simulink model "Induction_Motor"  (R2015a)
settings: Solver=FixedStepDiscrete  StartTime=0.0  StopTime=3  FixedStep=Ts  RelTol=1e-3
InitFcn:
  | Ts=1e-5;
values from neighbouring files (symbols this model uses):
  Mech_Load = 0.0    (= 0)    [runDistSim.m]    (also in run_all_dist_induction.m = [0.20, 0.80]*NominalTorque)
  Speed_Target = 1200    [runDistSim.m]    (also in run_all_dist_induction.m = 2240)
undefined symbols (not defined in the file or in its folder): ctrl_sat
libraries: powerlib x17, powerlib_extras x3, simulink x1, AC6DriveInternalModels x1
settings Model: Creator=Mademlis  LastModifiedBy=Savvas
settings DataIOCC: SignalLoggingSaveFormat=ModelDataLogs
settings OptimizationCC: ExpressionDepthLimit=2147483647
settings DebuggingCC: UnderspecifiedInitializationDetection=Classic  MergeDetectMultiDrivingBlocksExec=none  SolverPrmCheckMsg=warning  FcnCallInpInsideContextMsg=EnableAllAsWarning  StateNameClashWarn=warning

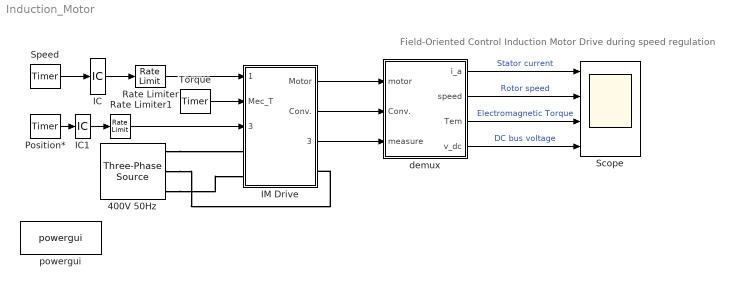
== system Induction_Motor ==
  note: Field-Oriented Control Induction Motor Drive during speed regulation
  400V 50Hz : powerlib/Electrical Sources/Three-Phase Source  Voltage=400  PhaseAngle=0  Frequency=50  InternalConnection=Yg  SpecifyImpedance=off  Resistance=0.02  Inductance=0.05e-3  ShortCircuitLevel=100e6  BaseVoltage=25e3  XRratio=7  BusType=swing  Pref=0  Qref=0  Qmin=-inf  Qmax=inf
  IC : InitialCondition  Value=0
  IC1 : InitialCondition  Value=0
  IM Drive : Subsystem
  Position* : powerlib_extras/Control  Blocks/Timer  t=[0 0.9]  e=[400 400]
  Rate Limiter : RateLimiter  RisingSlewLimit=600000  FallingSlewLimit=-600000  LinearizeAsGain=off
  Rate Limiter1 : RateLimiter  RisingSlewLimit=5000  FallingSlewLimit=-5000  LinearizeAsGain=off
  Scope : Scope  NumInputPorts=4
      settings: TimeRange=1.5  YMin=-28.89936~-296.83949~-32.87981~-120.93965  YMax=31.56272~1411.46172~57.70988~1089.39505  SaveName=simout  Decimation=25
  Speed : powerlib_extras/Control  Blocks/Timer  t=[0 0.1]  e=[0 Speed_Target]
  Torque : powerlib_extras/Control  Blocks/Timer  t=[0 0.6]  e=[0 Mech_Load]*10
  demux : Subsystem
  powergui : powerlib/powergui  Priority=2  SimulationMode=Discrete  SolverType=Tustin  SampleTime=Ts  frequency=60  SPID=off  DisableSnubberDevices=off  DisableRonSwitches=off  DisableVfSwitches=off  SwTol=0  DisplayEquations=off  Interpol=off  methode=off  Ts=0  FunctionMessages=off  echomessages=off  HookPort=off  EnableUseOfTLC=off  x0status=blocks  frequencyindice=50  Pbase=100e6  ErrMax=1e-4  Iterations=50  UnitsV=kV  UnitsW=MW  buscounter=0  RestoreLinks=warning  ResistiveCurrentMeasurement=off  Frange=[0:2:500]  Ylog=off  Xlog=on  ShowGrid=off  save=off  variable=ZData  structure=simout  ZoomFFT=on  StartTime=0.05  cycles=7  DisplayStyle=1  fundamental=60  FreqAxis=off  MaxFrequency=20000  frequencyindicesteady=1  RmsSteady=1  display=off
  wires:
  demux/1(i_a) -> Scope/1  "Stator current"
  demux/3(Tem) -> Scope/3  "Electromagnetic Torque"
  demux/4(v_dc) -> Scope/4  "DC bus voltage"
  demux/2(speed) -> Scope/2  "Rotor speed"
  Torque/1 -> IM Drive/2(Mec_T)
  Position*/1 -> IC1/1
  Rate Limiter/1 -> IM Drive/1(Speed*)
  Rate Limiter1/1 -> IM Drive/3(Position*)
  IC1/1 -> Rate Limiter1/1
  IM Drive/1(Motor) -> demux/1(motor)
  IM Drive/2(Conv.) -> demux/2(Conv.)
  IM Drive/3(measure) -> demux/3(measure)
  Speed/1 -> IC/1
  IC/1 -> Rate Limiter/1
  connections:
  400V 50Hz/RConn3 -- IM Drive/LConn2
  400V 50Hz/RConn1 -- IM Drive/LConn1
  400V 50Hz/RConn2 -- IM Drive/RConn1

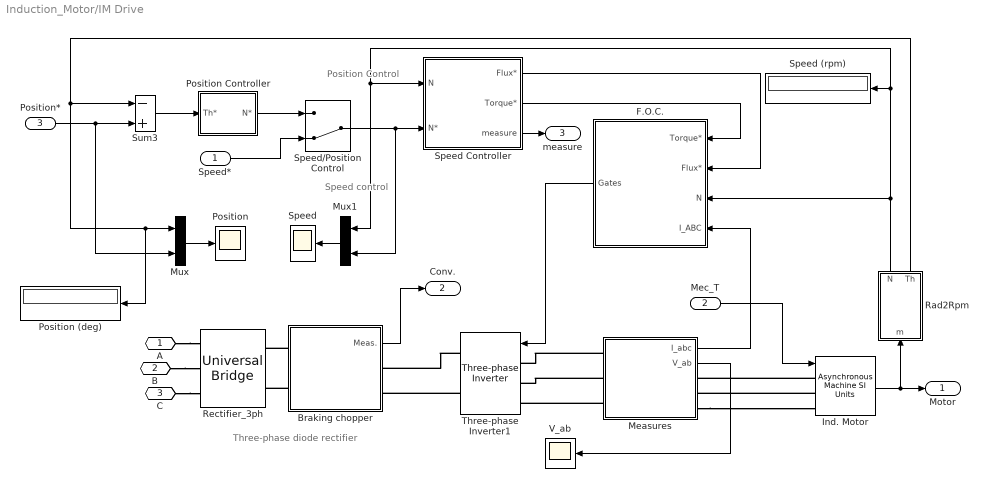
== system Induction_Motor/IM Drive ==
  note: Speed
      | control
  note: Position
      |  Control
  note: Three-phase
      | diode rectifier
  Speed* : Inport
  Mec_T : Inport  Port=2
  Position* : Inport  Port=3
  Braking chopper : Subsystem  mask(Braking chopper){chopa=650, chopd=530, freq_chop=1000, cap_bus=1500e-6, br=30}
      mask prompts: chopa "Chopper activation voltage (V)"; chopd "Chopper shutdown voltage (V)"; freq_chop "Braking chopper frequency (Hz)"; cap_bus "DC bus capacitance (F)"; br "Braking resistance (ohms)"
      mask help: This block implements a DC link between the rectifier and the inverter. It also contains a DC bus integrated braking chopper. The braking resistor must be set properly to avoid oscillation.
      mask init:
      | [X1,X1m,X2,X2m,X3,X4,Y1,Y1m,Y2,Y2m,Y3,Y4,color1,color2]=spsdrivelogo;
      mask Display:
      | patch([X1 X1m],[Y1 Y1m],color1);
      | patch(X3,Y3,color2);
      | plot([X1 X1m X2 X2m X3 X4],[Y1 Y1m Y2 Y2m Y3 Y4]);
  F.O.C. : Subsystem  mask(FOC){in_flux=0.85, Lm=0.50, Lls=0.027, Rr=3.2, Llr=0.027, p=2, Tvect=50e-6}
      mask prompts: in_flux "Initial machine flux (Wb)"; Lm "Motor mutual inductance (H)"; Lls "Motor stator Leakage inductance (H)"; Rr "Motor rotor resistance (ohms)"; Llr "Motor rotor leakage inductance (H)"; p "Motor pairs of poles"; Tvect "Vector control sampling time (s)"
      mask help: This block implements a field oriented controller.
      mask init:
      | Lr=Lm+Llr;
      | Ls=Lm+Lls;
      | [X1,X1m,X2,X2m,X3,X4,Y1,Y1m,Y2,Y2m,Y3,Y4,color1,color2]=spsdrivelogo;
      mask Display:
      | patch([X1 X1m],[Y1 Y1m],color1);
      | patch(X3,Y3,color2);
      | plot([X1 X1m X2 X2m X3 X4],[Y1 Y1m Y2 Y2m Y3 Y4]);
  Ind. Motor : powerlib/Machines/Asynchronous Machine SI Units  RotorType=Squirrel-cage  PresetModel=No  MechanicalLoad=Torque Tm  ShowDetailedParameters=on  ReferenceFrame=Rotor  Units=SI  MeasurementBus=off  NominalParameters=[2040 380 50]  Stator=[5.8 0.027]  Rotor=[3.2 0.027]  Cage1=[ 0.022 0.226/377]  Cage2=[ 0.022 0.226/377]  Lm=0.5  Mechanical=[0.047 0 2]  PolePairs=2  InitialConditions=[1 0 0 0 0 0 0 0]  SimulateSaturation=off  Saturation=[14.03593122, 27.81365428, 53.79336849, 72.68890987, 97.98006896, 148.6815601, 215.7428561, 302.9841135, 428.7778367 ; 230, 322, 414, 460, 506, 552, 598, 644, 690]  LoadFlowParameters=1492000  TsPowergui=0  TsBlock=-1  IterativeModel=Forward Euler  Pmec=1500
  Measures : Subsystem
  Mux : Mux  Inputs=2
  Mux1 : Mux  Inputs=2
  Position : Scope
      settings: YMin=-333.29346  YMax=2985.49263  SaveName=Angle
  Position (deg) : Display
  Position Controller : Subsystem  mask{Kp_th=2, T_position=5e-3}
      mask prompts: Kp_th "Proportional gain"; T_position "Controllersampling time (s)"
  Rad2Rpm : Subsystem
  Rectifier_3ph : powerlib/Power Electronics/Universal Bridge  Arms=3  SnubberResistance=10e3  SnubberCapacitance=20e-9  Device=Diodes  Ron=1e-3  Lon=0  ForwardVoltages="[  0,  0  ]"  ForwardVoltage=1.3  GTOparameters=[ 10e-6, 20e-6 ]  IGBTparameters=[ 1e-6 , 2e-6 ]  Measurements=All voltages and currents  Measurements_2=None  converterType=Rectifier
  Speed : Scope
      settings: TimeRange=1  YMin=-400  YMax=1400  SaveName=Speed_ref
  Speed (rpm) : Display
  Speed Controller : Subsystem  mask(Speed controller){kp=0.15, ki=0.0455, fc=50, ctrl_sat=[-30, 30], p=2, nf=0.85, Tsc=5e-3}
      mask prompts: kp "Proportional gain"; ki "Integral gain"; fc "Speed measurement - low-pass filter cutoff frequency (Hz)"; ctrl_sat "Controller output torque saturation (N.m) [negative,positive]"; p "Motor pairs of poles"; nf "Machine nominal flux (Wb)"; Tsc "Controller sampling time (s)"
      mask help: This block implements a PI speed regulator.
      mask init:
      | [X1,X1m,X2,X2m,X3,X4,Y1,Y1m,Y2,Y2m,Y3,Y4,color1,color2]=spsdrivelogo;
      mask Display:
      | patch([X1 X1m],[Y1 Y1m],color1);
      | patch(X3,Y3,color2);
      | plot([X1 X1m X2 X2m X3 X4],[Y1 Y1m Y2 Y2m Y3 Y4]);
  Speed/Position Control : ManualSwitch  CurrentSetting=0
  Sum3 : Sum  Inputs=-+  SaturateOnIntegerOverflow=on  InputSameDT=on  OutDataTypeStr=Inherit: Same as first input
  Three-phase Inverter1 : AC6DriveInternalModels/Three-phase Inverter  Arms=3  SnubberResistance=5000  SnubberCapacitance=inf  Device=IGBT / Diodes  Ron=1e-3  Lon=0  ForwardVoltages=[0.8,0.8]  ForwardVoltage=0  GTOparameters=[0,0]  IGBTParameters=[1e-6,2e-6]  Measurements=All voltages and currents  converterType=Inverter  SourceFrequency=60  dqInductances=[8.5e-3,8.5e-3]  Flux=0.175  Resistance=0.2  p=4
  V_ab : Scope
      settings: YMin=-50  YMax=50  SaveName=simout1
  A : PMIOPort  Port=1  Side=Left
  B : PMIOPort  Port=2  Side=Right
  C : PMIOPort  Port=3  Side=Left
  Motor : Outport
  Conv. : Outport  Port=2
  measure : Outport  Port=3
  wires:
  Mux1/1 -> Speed/1
  Measures/2(V_ab) -> V_ab/1
  Position*/1 -> Sum3/2, Mux/2
  Position Controller/1(N*) -> Speed/Position Control/1
  Speed/Position Control/1 -> Speed Controller/2(N*), Mux1/2
  Speed*/1 -> Speed/Position Control/2
  Sum3/1 -> Position Controller/1(Th*)
  Mux/1 -> Position/1
  Rad2Rpm/2(Th) -> Sum3/1, Mux/1, Position (deg)/1
  F.O.C./1(Gates) -> Three-phase Inverter1/1
  Braking chopper/1(Meas.) -> Conv./1
  Speed Controller/1(Flux*) -> F.O.C./2(Flux*)
  Speed Controller/3(measure) -> measure/1
  Ind. Motor/1 -> Motor/1, Rad2Rpm/1(m)
  Measures/1(I_abc) -> F.O.C./4(I_ABC)
  Speed Controller/2(Torque*) -> F.O.C./1(Torque*)
  Mec_T/1 -> Ind. Motor/1
  Rad2Rpm/1(N) -> Speed (rpm)/1, Speed Controller/1(N), Mux1/1, F.O.C./3(N)
  connections:
  C/RConn1 -- Rectifier_3ph/LConn3
  Braking chopper/LConn2 -- Rectifier_3ph/RConn2
  A/RConn1 -- Rectifier_3ph/LConn1
  Ind. Motor/LConn2 -- Measures/RConn2
  Ind. Motor/LConn1 -- Measures/RConn1
  Measures/LConn3 -- Three-phase Inverter1/LConn3
  Measures/RConn3 -- Ind. Motor/LConn3
  Three-phase Inverter1/RConn1 -- Braking chopper/RConn1
  Three-phase Inverter1/RConn2 -- Braking chopper/RConn2
  Braking chopper/LConn1 -- Rectifier_3ph/RConn1
  B/RConn1 -- Rectifier_3ph/LConn2
  Measures/LConn1 -- Three-phase Inverter1/LConn1
  Measures/LConn2 -- Three-phase Inverter1/LConn2

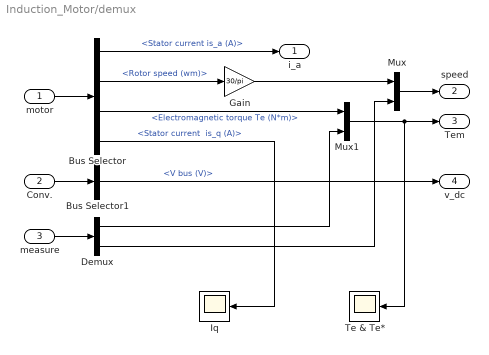
== system Induction_Motor/demux ==
  motor : Inport
  Conv. : Inport  Port=2
  measure : Inport  Port=3
  Bus Selector : BusSelector  OutputSignals="Stator measurements.Stator current is_a (A),Mechanical.Rotor speed (wm),Mechanical.Electromagnetic torque Te (N*m),Stator measurements.Stator current  is_q (A)"
  Bus Selector1 : BusSelector  OutputSignals=V bus (V)
  Demux : Demux  Outputs=2
  Gain : Gain  Gain=30/pi  SaturateOnIntegerOverflow=on  OutDataTypeStr=Inherit: Same as input  ParamDataTypeStr=Inherit: Same as input
  Iq : Scope
      settings: YMin=-50  YMax=50  SaveName=Torque1
  Mux : Mux  Inputs=2
  Mux1 : Mux  Inputs=2
  Te & Te* : Scope
      settings: YMin=-50  YMax=50  SaveName=Torque
  i_a : Outport
  speed : Outport  Port=2
  Tem : Outport  Port=3
  v_dc : Outport  Port=4
  wires:
  motor/1 -> Bus Selector/1
  Mux/1 -> speed/1
  Mux1/1 -> Tem/1, Te & Te*/1
  Bus Selector/3 -> Mux1/1  "<Electromagnetic torque Te (N*m)>"
  Bus Selector/2 -> Gain/1  "<Rotor speed (wm)>"
  Bus Selector/1 -> i_a/1  "<Stator current is_a (A)>"
  Gain/1 -> Mux/1
  Demux/2 -> Mux/2
  Demux/1 -> Mux1/2
  Conv./1 -> Bus Selector1/1
  Bus Selector1/1 -> v_dc/1  "<V bus (V)>"
  measure/1 -> Demux/1
  Bus Selector/4 -> Iq/1  "<Stator current  is_q (A)>"

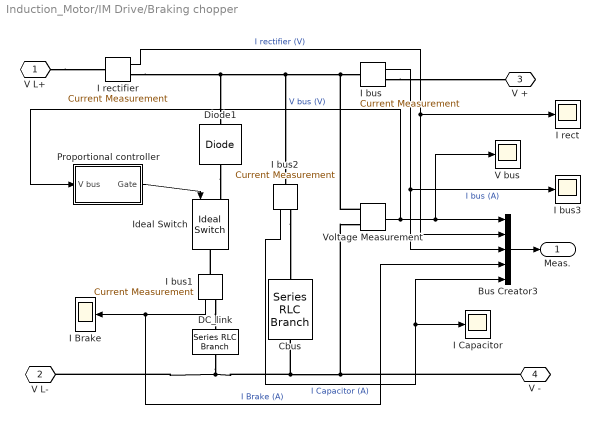
== system Induction_Motor/IM Drive/Braking chopper ==
  Bus Creator3 : BusCreator  Inputs=5
  Cbus : powerlib/Elements/Series RLC Branch  LConnTagsString=__new0  RConnTagsString=__new0  BranchType=C  Resistance=[]  Inductance=[]  SetiL0=off  InitialCurrent=0  Capacitance=cap_bus  Setx0=off  InitialVoltage=0  Measurements=None
  DC_link : powerlib/Elements/Series RLC Branch  LConnTagsString=__new0  RConnTagsString=__new0  BranchType=R  Resistance=br  Inductance=[]  SetiL0=off  InitialCurrent=0  Capacitance=[]  Setx0=off  InitialVoltage=0  Measurements=None
  Diode1 : powerlib/Power Electronics/Diode  Ron=0.01  Lon=0  Vf=0.8  IC=0  UseSnubber=off  Rs=10  Cs=10e-9  Measurements=off
  I Brake : Scope
      settings: YMin=-2.5  YMax=32.5  SaveName=I_brake
  I Capacitor : Scope
      settings: TimeRange=2  YMin=-200  YMax=200  SaveName=Ic
  I bus : powerlib/Measurements/Current Measurement  PhasorSimulation=off  OutputType=Complex  PSBequivalent=0
  I bus1 : powerlib/Measurements/Current Measurement  PhasorSimulation=off  OutputType=Complex  PSBequivalent=0
  I bus2 : powerlib/Measurements/Current Measurement  PhasorSimulation=off  OutputType=Complex  PSBequivalent=0
  I bus3 : Scope
      settings: YMin=0  YMax=950  SaveName=I_bus
  I rect : Scope
      settings: YMin=0  YMax=950  SaveName=I_rect
  I rectifier : powerlib/Measurements/Current Measurement  PhasorSimulation=off  OutputType=Complex  PSBequivalent=0
  Ideal Switch : powerlib/Power Electronics/Ideal Switch  Ron=0.01  Lon=0  IC=0  Rs=0.1  Cs=0.01e-6  Measurements=off
      settings: AttributesFormatString=\n
  Proportional controller : Subsystem
  V bus : Scope
      settings: TimeRange=2  YMin=0  YMax=950  SaveName=Vdc
  Voltage Measurement : powerlib/Measurements/Voltage Measurement  Tag=PoWeRsYsTeMmEaSuReMeNt  PhasorSimulation=off  OutputType=Complex  PSBequivalent=0
  V L+ : PMIOPort  Port=1  Side=Left
  V L- : PMIOPort  Port=2  Side=Left
  V + : PMIOPort  Port=3  Side=Right
  V - : PMIOPort  Port=4  Side=Right
  Meas. : Outport
  wires:
  Voltage Measurement/1 -> Bus Creator3/1, V bus/1, Proportional controller/1(V bus)  "V bus (V)"
  Proportional controller/1(Gate) -> Ideal Switch/1
  Bus Creator3/1 -> Meas./1
  I bus/1 -> Bus Creator3/3, I bus3/1  "I bus (A)"
  I rectifier/1 -> Bus Creator3/2, I rect/1  "I rectifier (V)"
  I bus1/1 -> I Brake/1, Bus Creator3/4  "I Brake (A)"
  I bus2/1 -> Bus Creator3/5, I Capacitor/1  "I Capacitor (A)"
  connections:
  Cbus/RConn1 -- V -/RConn1 -- Voltage Measurement/LConn2 -- V L-/RConn1 -- DC_link/RConn1
  Diode1/LConn1 -- I rectifier/RConn1 -- Voltage Measurement/LConn1 -- I bus/LConn1 -- I bus2/LConn1
  Diode1/RConn1 -- Ideal Switch/LConn1
  I bus/RConn1 -- V +/RConn1
  V L+/RConn1 -- I rectifier/LConn1
  I bus1/RConn1 -- DC_link/LConn1
  I bus1/LConn1 -- Ideal Switch/RConn1
  I bus2/RConn1 -- Cbus/LConn1

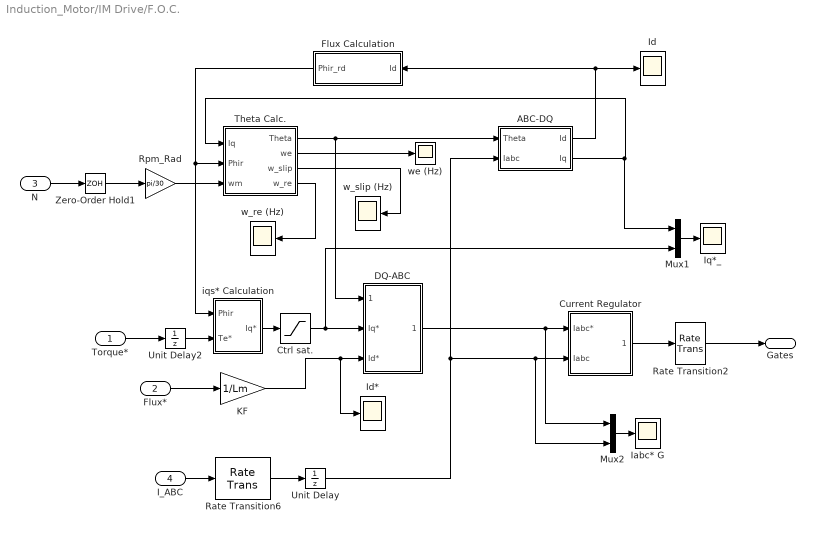
== system Induction_Motor/IM Drive/F.O.C. ==
  Torque* : Inport
  Flux* : Inport  Port=2
  N : Inport  Port=3
  I_ABC : Inport  Port=4
  ABC-DQ : Subsystem
  Ctrl sat. : Saturate  UpperLimit=26  LowerLimit=-26
  Current Regulator : Subsystem
  DQ-ABC : Subsystem
  Flux Calculation : Subsystem  mask(Flux Calcultation){}
      mask init:
      | NF=0.44572610323020e-6;
      | DF=[1 -0.99998715486734];
  Iabc* G : Scope
      settings: TimeRange=0.04  YMin=-30  YMax=30  SaveName=Iabc_G2
  Id : Scope
      settings: YMin=0  YMax=10  SaveName=Isd
  Id* : Scope
      settings: YMin=4.41347  YMax=4.87805  SaveName=Isd_ref
  Iq*_ : Scope
      settings: TimeRange=1  YMin=-20  YMax=30  SaveName=Iabc_G
  KF : Gain  Gain=1/Lm  SaturateOnIntegerOverflow=on  OutDataTypeStr=Inherit: Same as input  ParamDataTypeStr=Inherit: Same as input
  Mux1 : Mux  Inputs=2
  Mux2 : Mux  Inputs=2
  Rate Transition2 : RateTransition
  Rate Transition6 : RateTransition
  Rpm_Rad : Gain  Gain=pi/30  SaturateOnIntegerOverflow=on  OutDataTypeStr=Inherit: Same as input  ParamDataTypeStr=Inherit: Same as input
  Theta Calc. : Subsystem
  Unit Delay : UnitDelay  SampleTime=Tvect
  Unit Delay2 : UnitDelay  SampleTime=Tvect
  Zero-Order Hold1 : ZeroOrderHold  SampleTime=Tvect
  iqs* Calculation : Subsystem
  w_re (Hz) : Scope
      settings: YMin=0  YMax=100  SaveName=W_re_Hz
  w_slip (Hz) : Scope
      settings: YMin=0  YMax=100  SaveName=W_slip_Hz
  we (Hz) : Scope
      settings: YMin=-700  YMax=800  SaveName=we_Hz
  Gates : Outport
  wires:
  Mux2/1 -> Iabc* G/1
  Current Regulator/1(Pulses) -> Rate Transition2/1
  KF/1 -> DQ-ABC/3(Id*), Id*/1
  Flux*/1 -> KF/1
  iqs* Calculation/1(Iq*) -> Ctrl sat./1
  Rpm_Rad/1 -> Theta Calc./3(wm)
  ABC-DQ/1(Id) -> Id/1, Flux Calculation/1(Id)
  ABC-DQ/2(Iq) -> Mux1/1, Theta Calc./1(Iq)
  Flux Calculation/1(Phir_rd) -> iqs* Calculation/1(Phir), Theta Calc./2(Phir)
  Theta Calc./1(Theta) -> DQ-ABC/1(Theta), ABC-DQ/1(Theta)
  I_ABC/1 -> Rate Transition6/1
  Unit Delay/1 -> ABC-DQ/2(Iabc), Mux2/2, Current Regulator/2(Iabc)
  Torque*/1 -> Unit Delay2/1
  DQ-ABC/1(Iabc*) -> Mux2/1, Current Regulator/1(Iabc*)
  Rate Transition2/1 -> Gates/1
  Unit Delay2/1 -> iqs* Calculation/2(Te*)
  Rate Transition6/1 -> Unit Delay/1
  Theta Calc./2(we) -> we (Hz)/1
  Theta Calc./3(w_slip) -> w_slip (Hz)/1
  Theta Calc./4(w_re) -> w_re (Hz)/1
  Ctrl sat./1 -> Mux1/2, DQ-ABC/2(Iq*)
  Zero-Order Hold1/1 -> Rpm_Rad/1
  N/1 -> Zero-Order Hold1/1
  Mux1/1 -> Iq*_/1

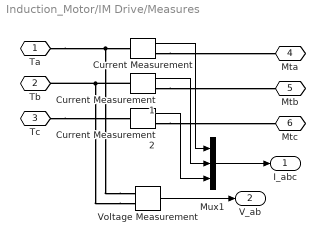
== system Induction_Motor/IM Drive/Measures ==
  Current Measurement : powerlib/Measurements/Current Measurement  Tag=PoWeRsYsTeMmEaSuReMeNt  PhasorSimulation=off  OutputType=Complex  PSBequivalent=0
  Current Measurement1 : powerlib/Measurements/Current Measurement  Tag=PoWeRsYsTeMmEaSuReMeNt  PhasorSimulation=off  OutputType=Complex  PSBequivalent=0
  Current Measurement2 : powerlib/Measurements/Current Measurement  Tag=PoWeRsYsTeMmEaSuReMeNt  PhasorSimulation=off  OutputType=Complex  PSBequivalent=0
  Mux1 : Mux  Inputs=3
  Voltage Measurement : powerlib/Measurements/Voltage Measurement  PhasorSimulation=off  OutputType=Complex  PSBequivalent=0
  Ta : PMIOPort  Port=1  Side=Left
  Tb : PMIOPort  Port=2  Side=Left
  Tc : PMIOPort  Port=3  Side=Left
  Mta : PMIOPort  Port=4  Side=Right
  Mtb : PMIOPort  Port=5  Side=Right
  Mtc : PMIOPort  Port=6  Side=Right
  I_abc : Outport
  V_ab : Outport  Port=2
  wires:
  Mux1/1 -> I_abc/1
  Current Measurement1/1 -> Mux1/2
  Current Measurement/1 -> Mux1/1
  Current Measurement2/1 -> Mux1/3
  Voltage Measurement/1 -> V_ab/1
  connections:
  Current Measurement1/RConn1 -- Mtb/RConn1
  Voltage Measurement/LConn2 -- Current Measurement1/LConn1 -- Tb/RConn1
  Current Measurement/RConn1 -- Mta/RConn1
  Voltage Measurement/LConn1 -- Ta/RConn1 -- Current Measurement/LConn1
  Tc/RConn1 -- Current Measurement2/LConn1
  Current Measurement2/RConn1 -- Mtc/RConn1

== system Induction_Motor/IM Drive/Position Controller ==
  Th* : Inport
  Discrete Derivative : simulink/Discrete/Discrete Derivative  gainval=1.0  ICPrevScaledInput=0.0  InputProcessing=Inherited  OutMin=[]  OutMax=[]  OutDataType=fixdt(1, 16)  OutScaling=2^-10  DoSatur=off
  Discrete-Time Integrator2 : DiscreteIntegrator  SampleTime=-1  UpperSaturationLimit=ctrl_sat(2)/3  LowerSaturationLimit=ctrl_sat(1)/3
  Integral gain : Gain  Gain=0  SampleTime=T_position  SaturateOnIntegerOverflow=on  OutDataTypeStr=Inherit: Same as input  ParamDataTypeStr=Inherit: Same as input
  Rate Transition1 : RateTransition
  Rate Transition2 : RateTransition
  Sum2 : Sum  Inputs=+++  SaturateOnIntegerOverflow=on  InputSameDT=on  OutDataTypeStr=Inherit: Same as first input
  kp_Th : Gain  Gain=Kp_th  SampleTime=T_position  SaturateOnIntegerOverflow=on  OutDataTypeStr=Inherit: Same as input  ParamDataTypeStr=Inherit: Same as input
  kp_Th1 : Gain  Gain=0  SampleTime=T_position  SaturateOnIntegerOverflow=on  OutDataTypeStr=Inherit: Same as input  ParamDataTypeStr=Inherit: Same as input
  N* : Outport
  wires:
  Th*/1 -> Rate Transition2/1
  Sum2/1 -> Rate Transition1/1
  Integral gain/1 -> Discrete-Time Integrator2/1
  Discrete Derivative/1 -> Sum2/3
  kp_Th/1 -> Sum2/2
  Discrete-Time Integrator2/1 -> Sum2/1
  kp_Th1/1 -> Discrete Derivative/1
  Rate Transition1/1 -> N*/1
  Rate Transition2/1 -> kp_Th/1, Integral gain/1, kp_Th1/1

== system Induction_Motor/IM Drive/Rad2Rpm ==
  m : Inport
  Demux : Demux  Outputs=[19 1 1 1]
  Rad/s2Rpm : Gain  Gain=30/pi  SaturateOnIntegerOverflow=on  OutDataTypeStr=Inherit: Same as input  ParamDataTypeStr=Inherit: Same as input
  Rad2deg : Gain  Gain=180/pi  SaturateOnIntegerOverflow=on  OutDataTypeStr=Inherit: Same as input  ParamDataTypeStr=Inherit: Same as input
  Terminator : Terminator
  Terminator1 : Terminator
  N : Outport
  Th : Outport  Port=2
  wires:
  Demux/1 -> Terminator1/1
  Demux/3 -> Terminator/1
  Demux/2 -> Rad/s2Rpm/1
  m/1 -> Demux/1
  Demux/4 -> Rad2deg/1
  Rad2deg/1 -> Th/1
  Rad/s2Rpm/1 -> N/1

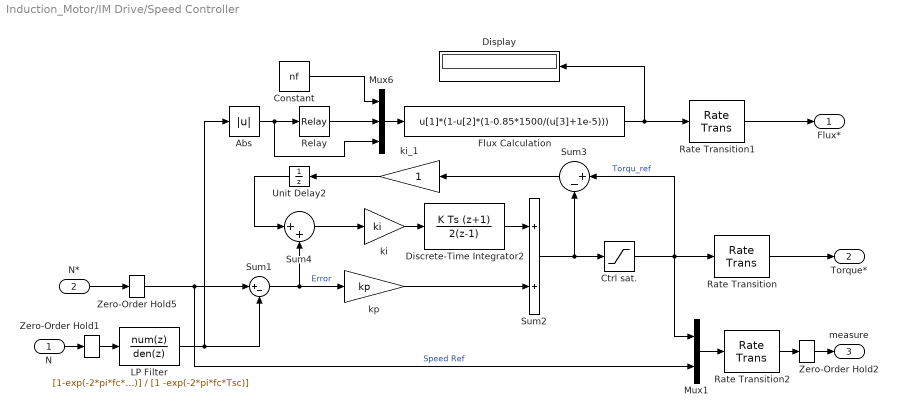
== system Induction_Motor/IM Drive/Speed Controller ==
  N : Inport
  N* : Inport  Port=2
  Abs : Abs  SaturateOnIntegerOverflow=on
  Constant : Constant  Value=nf
  Ctrl sat. : Saturate  UpperLimit=ctrl_sat(2)  LowerLimit=ctrl_sat(1)
  Discrete-Time Integrator2 : DiscreteIntegrator  IntegratorMethod=Integration: Trapezoidal  InitialConditionSetting=State (most efficient)  SampleTime=Tsc  LimitOutput=on  UpperSaturationLimit=ctrl_sat(2)/1  LowerSaturationLimit=ctrl_sat(1)/1
  Display : Display
  Flux Calculation : Fcn  Expr=u[1]*(1-u[2]*(1-0.85*1500/(u[3]+1e-5)))
  LP Filter : DiscreteTransferFcn  Numerator=[1-exp(-2*pi*fc*Tsc)]  Denominator=[1 -exp(-2*pi*fc*Tsc)]  SampleTime=Tsc
  Mux1 : Mux  Inputs=2
  Mux6 : Mux  Inputs=3
  Rate Transition : RateTransition
  Rate Transition1 : RateTransition
  Rate Transition2 : RateTransition
  Relay : Relay  OnSwitchValue=1500  OffSwitchValue=1500
  Sum1 : Sum  Inputs=|+-  SaturateOnIntegerOverflow=on  InputSameDT=on  OutDataTypeStr=Inherit: Same as first input
  Sum2 : Sum  SaturateOnIntegerOverflow=on  InputSameDT=on  OutDataTypeStr=Inherit: Same as first input
  Sum3 : Sum  Inputs=|+-
  Sum4 : Sum  Inputs=|++
  Unit Delay2 : UnitDelay  SampleTime=-1
  Zero-Order Hold1 : ZeroOrderHold  SampleTime=Tsc
  Zero-Order Hold2 : ZeroOrderHold  SampleTime=Ts
  Zero-Order Hold5 : ZeroOrderHold  SampleTime=Tsc
  ki : Gain  Gain=ki  SaturateOnIntegerOverflow=on  OutDataTypeStr=Inherit: Same as input  ParamDataTypeStr=Inherit: Same as input
  ki_1 : Gain  SaturateOnIntegerOverflow=on  OutDataTypeStr=Inherit: Same as input  ParamDataTypeStr=Inherit: Same as input
  kp : Gain  Gain=kp  SaturateOnIntegerOverflow=on  OutDataTypeStr=Inherit: Same as input  ParamDataTypeStr=Inherit: Same as input
  Flux* : Outport
  Torque* : Outport  Port=2
  measure : Outport  Port=3
  wires:
  Zero-Order Hold2/1 -> measure/1
  Discrete-Time Integrator2/1 -> Sum2/1
  Zero-Order Hold1/1 -> LP Filter/1
  Zero-Order Hold5/1 -> Sum1/1, Mux1/2  "Speed Ref"
  Rate Transition1/1 -> Flux*/1
  Mux1/1 -> Rate Transition2/1
  Rate Transition2/1 -> Zero-Order Hold2/1
  Rate Transition/1 -> Torque*/1
  kp/1 -> Sum2/2
  N/1 -> Zero-Order Hold1/1
  Sum1/1 -> kp/1, Sum4/2  "Error"
  ki/1 -> Discrete-Time Integrator2/1
  LP Filter/1 -> Sum1/2, Abs/1
  Sum2/1 -> Ctrl sat./1, Sum3/2
  Ctrl sat./1 -> Rate Transition/1, Mux1/1, Sum3/1  "Torqu_ref"
  N*/1 -> Zero-Order Hold5/1
  Flux Calculation/1 -> Display/1, Rate Transition1/1
  Abs/1 -> Relay/1, Mux6/3
  Constant/1 -> Mux6/1
  Relay/1 -> Mux6/2
  Mux6/1 -> Flux Calculation/1
  Sum4/1 -> ki/1
  Sum3/1 -> ki_1/1
  ki_1/1 -> Unit Delay2/1
  Unit Delay2/1 -> Sum4/1

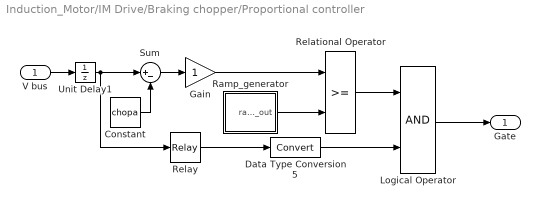
== system Induction_Motor/IM Drive/Braking chopper/Proportional controller ==
  V bus : Inport
  Constant : Constant  Value=chopa
  Data Type Conversion5 : DataTypeConversion  SaturateOnIntegerOverflow=on  RndMeth=Zero
  Gain : Gain  SaturateOnIntegerOverflow=on  OutDataTypeStr=Inherit: Same as input  ParamDataTypeStr=Inherit: Same as input
  Logical Operator : Logic
  Ramp_generator : Subsystem
  Relational Operator : RelationalOperator  InputSameDT=on
  Relay : Relay  OnSwitchValue=chopa  OffSwitchValue=chopd
  Sum : Sum  Inputs=|+-  SaturateOnIntegerOverflow=on  InputSameDT=on  OutDataTypeStr=Inherit: Same as first input
  Unit Delay1 : UnitDelay  SampleTime=Ts
  Gate : Outport
  wires:
  Data Type Conversion5/1 -> Logical Operator/2
  Relay/1 -> Data Type Conversion5/1
  Logical Operator/1 -> Gate/1
  Relational Operator/1 -> Logical Operator/1
  V bus/1 -> Unit Delay1/1
  Constant/1 -> Sum/2
  Gain/1 -> Relational Operator/1
  Sum/1 -> Gain/1
  Unit Delay1/1 -> Relay/1, Sum/1
  Ramp_generator/1(ramp_out) -> Relational Operator/2

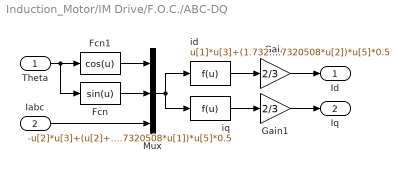
== system Induction_Motor/IM Drive/F.O.C./ABC-DQ ==
  Theta : Inport
  Iabc : Inport  Port=2
  Fcn : Fcn  Expr=sin(u)
  Fcn1 : Fcn  Expr=cos(u)
  Gain : Gain  Gain=2/3  SaturateOnIntegerOverflow=on  OutDataTypeStr=Inherit: Same as input  ParamDataTypeStr=Inherit: Same as input
  Gain1 : Gain  Gain=2/3  SaturateOnIntegerOverflow=on  OutDataTypeStr=Inherit: Same as input  ParamDataTypeStr=Inherit: Same as input
  Mux : Mux  Inputs=[1 1 3]
  id : Fcn  Expr=u[1]*u[3]+(1.7320508*u[2]-u[1])*u[4]*0.5+(-u[1]-1.7320508*u[2])*u[5]*0.5
  iq : Fcn  Expr=-u[2]*u[3]+(u[2]+1.7320508*u[1])*u[4]*0.5+(u[2]-1.7320508*u[1])*u[5]*0.5
  Id : Outport  InitialOutput=0
  Iq : Outport  Port=2  InitialOutput=0
  wires:
  Fcn/1 -> Mux/2
  Fcn1/1 -> Mux/1
  Theta/1 -> Fcn1/1, Fcn/1
  Mux/1 -> iq/1, id/1
  Iabc/1 -> Mux/3
  iq/1 -> Gain1/1
  id/1 -> Gain/1
  Gain/1 -> Id/1
  Gain1/1 -> Iq/1

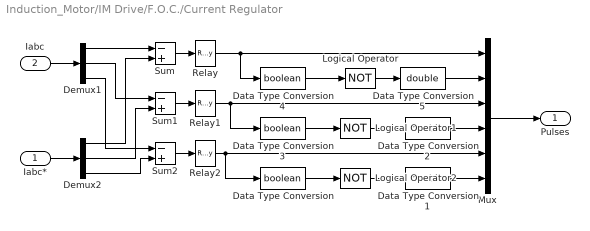
== system Induction_Motor/IM Drive/F.O.C./Current Regulator ==
  Iabc* : Inport
  Iabc : Inport  Port=2
  Data Type Conversion : DataTypeConversion  OutDataTypeStr=boolean  SaturateOnIntegerOverflow=on  RndMeth=Zero
  Data Type Conversion1 : DataTypeConversion  OutDataTypeStr=double  SaturateOnIntegerOverflow=on  RndMeth=Zero
  Data Type Conversion2 : DataTypeConversion  OutDataTypeStr=double  SaturateOnIntegerOverflow=on  RndMeth=Zero
  Data Type Conversion3 : DataTypeConversion  OutDataTypeStr=boolean  SaturateOnIntegerOverflow=on  RndMeth=Zero
  Data Type Conversion4 : DataTypeConversion  OutDataTypeStr=boolean  SaturateOnIntegerOverflow=on  RndMeth=Zero
  Data Type Conversion5 : DataTypeConversion  OutDataTypeStr=double  SaturateOnIntegerOverflow=on  RndMeth=Zero
  Demux1 : Demux  Outputs=3
  Demux2 : Demux  Outputs=3
  Logical Operator : Logic  Operator=NOT
  Logical Operator1 : Logic  Operator=NOT
  Logical Operator2 : Logic  Operator=NOT
  Mux : Mux  Inputs=6
  Relay : Relay  OnSwitchValue=0  OffSwitchValue=0
  Relay1 : Relay  OnSwitchValue=0  OffSwitchValue=0
  Relay2 : Relay  OnSwitchValue=0  OffSwitchValue=0
  Sum : Sum  Inputs=-+  SaturateOnIntegerOverflow=on  InputSameDT=on  OutDataTypeStr=Inherit: Same as first input
  Sum1 : Sum  Inputs=-+  SaturateOnIntegerOverflow=on  InputSameDT=on  OutDataTypeStr=Inherit: Same as first input
  Sum2 : Sum  Inputs=-+  SaturateOnIntegerOverflow=on  InputSameDT=on  OutDataTypeStr=Inherit: Same as first input
  Pulses : Outport  InitialOutput=0
  wires:
  Data Type Conversion5/1 -> Mux/2
  Data Type Conversion4/1 -> Logical Operator/1
  Data Type Conversion3/1 -> Logical Operator1/1
  Data Type Conversion2/1 -> Mux/4
  Data Type Conversion1/1 -> Mux/6
  Data Type Conversion/1 -> Logical Operator2/1
  Sum/1 -> Relay/1
  Sum1/1 -> Relay1/1
  Demux1/1 -> Sum/1
  Demux1/2 -> Sum1/1
  Mux/1 -> Pulses/1
  Iabc/1 -> Demux1/1
  Sum2/1 -> Relay2/1
  Demux1/3 -> Sum2/1
  Demux2/3 -> Sum2/2
  Demux2/2 -> Sum1/2
  Demux2/1 -> Sum/2
  Iabc*/1 -> Demux2/1
  Relay/1 -> Data Type Conversion4/1, Mux/1
  Relay1/1 -> Data Type Conversion3/1, Mux/3
  Relay2/1 -> Data Type Conversion/1, Mux/5
  Logical Operator/1 -> Data Type Conversion5/1
  Logical Operator1/1 -> Data Type Conversion2/1
  Logical Operator2/1 -> Data Type Conversion1/1

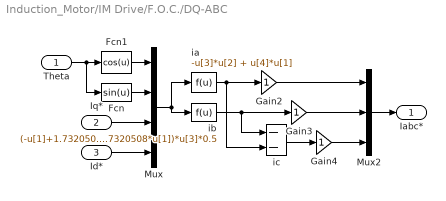
== system Induction_Motor/IM Drive/F.O.C./DQ-ABC ==
  Theta : Inport
  Iq* : Inport  Port=2
  Id* : Inport  Port=3
  Fcn : Fcn  Expr=sin(u)
  Fcn1 : Fcn  Expr=cos(u)
  Gain2 : Gain  SaturateOnIntegerOverflow=on  OutDataTypeStr=Inherit: Same as input  ParamDataTypeStr=Inherit: Same as input
  Gain3 : Gain  SaturateOnIntegerOverflow=on  OutDataTypeStr=Inherit: Same as input  ParamDataTypeStr=Inherit: Same as input
  Gain4 : Gain  SaturateOnIntegerOverflow=on  OutDataTypeStr=Inherit: Same as input  ParamDataTypeStr=Inherit: Same as input
  Mux : Mux
  Mux2 : Mux  Inputs=3
  ia : Fcn  Expr=-u[3]*u[2] + u[4]*u[1]
  ib : Fcn  Expr=(-u[1]+1.7320508*u[2])*u[4]*0.5+(u[2]+1.7320508*u[1])*u[3]*0.5
  ic : Sum  Inputs=--  SaturateOnIntegerOverflow=on  InputSameDT=on  OutDataTypeStr=Inherit: Same as first input
  Iabc* : Outport  InitialOutput=0
  wires:
  Fcn/1 -> Mux/2
  Fcn1/1 -> Mux/1
  Mux2/1 -> Iabc*/1
  Mux/1 -> ib/1, ia/1
  Theta/1 -> Fcn1/1, Fcn/1
  Iq*/1 -> Mux/3
  Id*/1 -> Mux/4
  Gain3/1 -> Mux2/2
  ic/1 -> Gain4/1
  Gain4/1 -> Mux2/3
  Gain2/1 -> Mux2/1
  ia/1 -> Gain2/1, ic/2
  ib/1 -> Gain3/1, ic/1

== system Induction_Motor/IM Drive/F.O.C./Flux Calculation ==
  note: Phir = Lm *Id / (1 +Tr .s)
  Id : Inport
  Discrete Transfer Fcn1 : DiscreteTransferFcn  Numerator=[1-exp(-(Rr/(Lr))*Tvect)]  Denominator=[1 -exp(-(Rr/(Lr))*Tvect)]  SampleTime=Tvect
  Lm : Gain  Gain=Lm  SaturateOnIntegerOverflow=on  OutDataTypeStr=Inherit: Same as input  ParamDataTypeStr=Inherit: Same as input
  Phir_rd : Outport
  wires:
  Discrete Transfer Fcn1/1 -> Phir_rd/1
  Id/1 -> Lm/1
  Lm/1 -> Discrete Transfer Fcn1/1

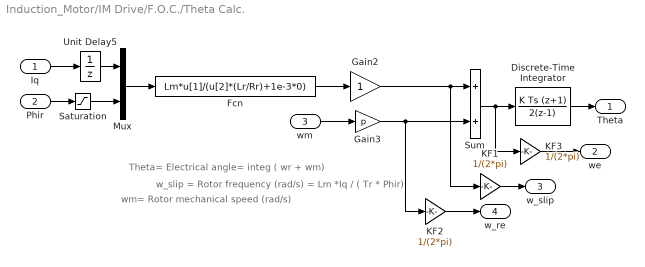
== system Induction_Motor/IM Drive/F.O.C./Theta Calc. ==
  note: Theta= Electrical angle= integ ( wr + wm)
  note: w_slip = Rotor frequency (rad/s) = Lm *Iq / ( Tr * Phir)
  note: wm= Rotor mechanical speed (rad/s)
  Iq : Inport
  Phir : Inport  Port=2
  wm : Inport  Port=3
  Discrete-Time Integrator : DiscreteIntegrator  IntegratorMethod=Integration: Trapezoidal  SampleTime=Tvect
  Fcn : Fcn  Expr=Lm*u[1]/(u[2]*(Lr/Rr)+1e-3*0)
  Gain2 : Gain  SaturateOnIntegerOverflow=on  OutDataTypeStr=Inherit: Same as input  ParamDataTypeStr=Inherit: Same as input
  Gain3 : Gain  Gain=p  SaturateOnIntegerOverflow=on  OutDataTypeStr=Inherit: Same as input  ParamDataTypeStr=Inherit: Same as input
  KF1 : Gain  Gain=1/(2*pi)  SaturateOnIntegerOverflow=on  OutDataTypeStr=Inherit: Same as input  ParamDataTypeStr=Inherit: Same as input
  KF2 : Gain  Gain=1/(2*pi)  SaturateOnIntegerOverflow=on  OutDataTypeStr=Inherit: Same as input  ParamDataTypeStr=Inherit: Same as input
  KF3 : Gain  Gain=1/(2*pi)  SaturateOnIntegerOverflow=on  OutDataTypeStr=Inherit: Same as input  ParamDataTypeStr=Inherit: Same as input
  Mux : Mux  Inputs=2
  Saturation : Saturate  UpperLimit=inf  LowerLimit=1e-3
  Sum : Sum  SaturateOnIntegerOverflow=on  InputSameDT=on  OutDataTypeStr=Inherit: Same as first input
  Unit Delay5 : UnitDelay  SampleTime=Tvect
  Theta : Outport  InitialOutput=0
  we : Outport  Port=2  InitialOutput=0
  w_slip : Outport  Port=3  InitialOutput=0
  w_re : Outport  Port=4  InitialOutput=0
  wires:
  Discrete-Time Integrator/1 -> Theta/1
  Sum/1 -> Discrete-Time Integrator/1, KF3/1
  Gain3/1 -> Sum/2, KF2/1
  Gain2/1 -> Sum/1, KF1/1
  wm/1 -> Gain3/1
  Fcn/1 -> Gain2/1
  Phir/1 -> Saturation/1
  Iq/1 -> Unit Delay5/1
  Mux/1 -> Fcn/1
  Saturation/1 -> Mux/2
  Unit Delay5/1 -> Mux/1
  KF1/1 -> w_slip/1
  KF2/1 -> w_re/1
  KF3/1 -> we/1

== system Induction_Motor/IM Drive/F.O.C./iqs* Calculation ==
  Phir : Inport
  Te* : Inport  Port=2
  Fcn : Fcn  Expr=(2/3)*(1/p)*(Lr/Lm)*u[1]/(u[2]+1e-3*0)
  Mux1 : Mux  Inputs=2
  Saturation : Saturate  UpperLimit=inf  LowerLimit=1e-3
  Iq* : Outport  InitialOutput=0
  wires:
  Phir/1 -> Saturation/1
  Fcn/1 -> Iq*/1
  Te*/1 -> Mux1/1
  Mux1/1 -> Fcn/1
  Saturation/1 -> Mux1/2

== system Induction_Motor/IM Drive/Braking chopper/Proportional controller/Ramp_generator ==
  Constant3 : Constant
  Discrete-Time Integrator1 : DiscreteIntegrator  ExternalReset=rising  SampleTime=Ts
  Relational Operator1 : RelationalOperator  InputSameDT=on
  Unit Delay1 : UnitDelay  SampleTime=Ts
  fc : Constant  Value=freq_chop
  ramp_out : Outport
  wires:
  Unit Delay1/1 -> Discrete-Time Integrator1/2
  Relational Operator1/1 -> Unit Delay1/1
  Constant3/1 -> Relational Operator1/2
  Discrete-Time Integrator1/1 -> ramp_out/1, Relational Operator1/1
  fc/1 -> Discrete-Time Integrator1/1
